simulink model "continous_model"  (R2017b)
settings: Solver=VariableStepAuto  StartTime=0.0  StopTime=70  RelTol=1e-3
values from neighbouring files (symbols this model uses):
  a1 = 0.44    [workspace.mat]    (also in workspace2.mat)
  a2 = 0.51    [workspace.mat]    (also in workspace2.mat)
  a3 = 0.48    [workspace.mat]    (also in workspace2.mat)
  a4 = -0.65    [workspace.mat]    (also in workspace2.mat)
  K = 2.5    [workspace.mat]    (also in workspace2.mat)
  T1 = 5    [workspace.mat]    (also in workspace2.mat)
  T2 = 10    [workspace.mat]    (also in workspace2.mat)
settings Model: Creator=gulin  LastModifiedBy=gulin

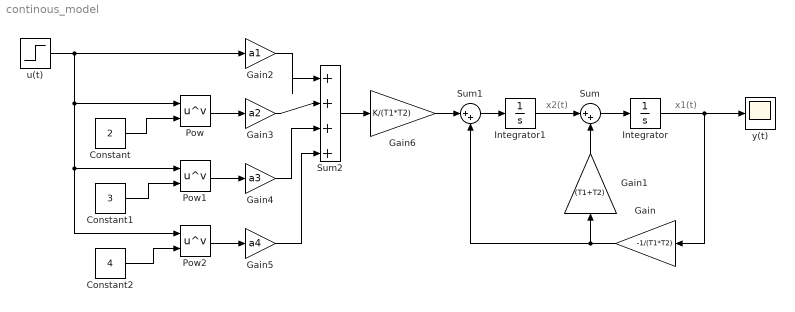
== system continous_model ==
  note: x1(t)
  note: x2(t)
  Constant : Constant  Value=2
  Constant1 : Constant  Value=3
  Constant2 : Constant  Value=4
  Gain : Gain  Gain=-1/(T1*T2)
  Gain1 : Gain  Gain=(T1+T2)
  Gain2 : Gain  Gain=a1
  Gain3 : Gain  Gain=a2
  Gain4 : Gain  Gain=a3
  Gain5 : Gain  Gain=a4
  Gain6 : Gain  Gain=K/(T1*T2)
  Integrator : Integrator
  Integrator1 : Integrator
  Pow : Math  Operator=pow  RndMeth=Zero  SaturateOnIntegerOverflow=on
  Pow1 : Math  Operator=pow  RndMeth=Zero  SaturateOnIntegerOverflow=on
  Pow2 : Math  Operator=pow  RndMeth=Zero  SaturateOnIntegerOverflow=on
  Sum : Sum  Inputs=|++
  Sum1 : Sum  Inputs=|++
  Sum2 : Sum  Inputs=|++++
  "u(t) " : Step  SampleTime=0
  "y(t) " : Scope
  wires:
  Sum/1 -> Integrator/1
  Integrator/1 -> Gain/1, "y(t) "/1
  Gain/1 -> Gain1/1, Sum1/2
  Integrator1/1 -> Sum/1
  Sum1/1 -> Integrator1/1
  Gain1/1 -> Sum/2
  Gain5/1 -> Sum2/4
  Gain4/1 -> Sum2/3
  Gain3/1 -> Sum2/2
  Gain2/1 -> Sum2/1
  Sum2/1 -> Gain6/1
  Gain6/1 -> Sum1/1
  Pow/1 -> Gain3/1
  "u(t) "/1 -> Pow2/1, Pow1/1, Pow/1, Gain2/1
  Pow1/1 -> Gain4/1
  Pow2/1 -> Gain5/1
  Constant/1 -> Pow/2
  Constant1/1 -> Pow1/2
  Constant2/1 -> Pow2/2
